simulink model "BalekaTorqueRamp"  (R2025a)
settings: Solver=FixedStepAuto  StartTime=0.0  StopTime=StopTime  RelTol=1e-3
values from neighbouring files (symbols this model uses):
  StopTime = 15    [StepParams.m]
undefined symbols (not defined in the file or in its folder): HS, IO291
libraries: aru_toolbox x7, simulink x4, speedgoatlib_IO691 x3, speedgoatlib_IO291 x1
settings Model: SimulationMode=external  Creator=Blue Fifth  LastModifiedBy=user
settings SolverCC: ConcurrentTasks=on  PositivePriorityOrder=on
settings OptimizationCC: BlockReduction=off  OptimizeBlockIOStorage=off
settings DebuggingCC: TasksWithSamePriorityMsg=none
settings HardwareCC: ProdBitPerLong=64.0  ProdLongLongMode=on  ProdHWDeviceType=Intel->x86-64 (Linux 64)
settings RTWCC: SystemTargetFile=speedgoat.tlc  TemplateMakefile=slrealtime_default_tmf  Toolchain=Simulink Real-Time Toolchain  BuildConfiguration=Faster Runs  CodeExecutionProfiling=on  TargetLang=C++  GPUComputeCapability=3.5  Description=Speedgoat Real-Time Target Machine
settings SimulinkRealTimeTargetCC: SLRTFileLogMaxRuns=1.0  ExtModeMaxTrigDuration=10.0  ExtModeStaticAllocSize=1000000.0  ExtModeTransport=0.0  MultiwordLength=2048.0  DynamicStringBufferSize=256.0  PreserveMATLABNamespacesInGeneratedCode=on  SubcomponentCodeInterfacePackaging=Reusable function  InstructionSetFMA=off  LogToMDFFile=off

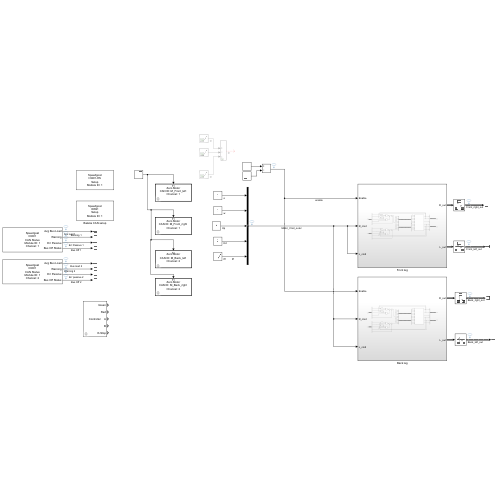
[thumbnail: Simulink's stored preview of the top-level diagram]
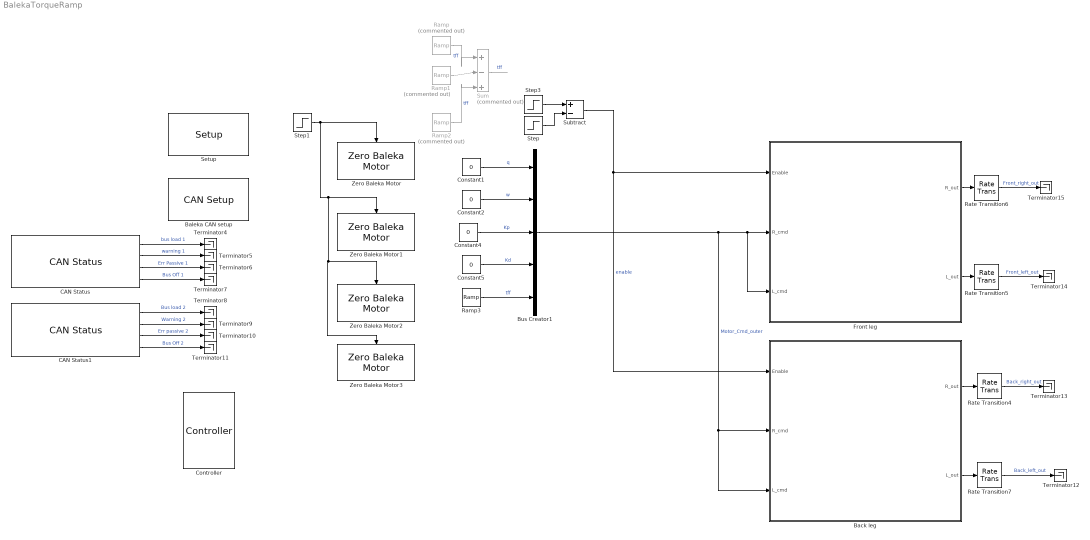
== system BalekaTorqueRamp ==
  Back leg : Subsystem
  Baleka CAN setup : speedgoatlib_IO691/Legacy/CAN Setup   moduletype=IO691  id=1  pciSlot=-1  chn1=CAN (HS)  chn2=CAN (HS)  chn3=Disabled  chn4=Disabled  initStruct=[]  termStruct=[struct('Channel',1,'Protocol','CAN','BRS',0,'Type','Extended','Identifier',1,'Data',[255, 255, 255, 255, 255, 255, 255, 253],'Pause',0.001), struct('Channel',2,'Protocol','CAN','BRS',0,'Type','Extended','Identifier',2,'Data',[255, 255, 255, 255, 255, 255, 255, 253],'Pause',0.001)]  ArbitrationbdrChn1=1.0 MBaud  ArbitrationManbdrChn1=[2,8,31,8]  FdbdrChn1=1.0 MBaud  FdManbdrChn1=[2,8,31,8]  ArbitrationbdrChn2=1.0 MBaud  ArbitrationManbdrChn2=[2,8,31,8]  FdbdrChn2=1.0 MBaud  FdManbdrChn2=[2,8,31,8]  ArbitrationbdrChn3=1.0 MBaud  ArbitrationManbdrChn3=[2,8,31,8]  FdbdrChn3=5.0 MBaud  FdManbdrChn3=[2,2,5,2]  ArbitrationbdrChn4=1.0 MBaud  ArbitrationManbdrChn4=[2,8,31,8]  FdbdrChn4=5.0 MBaud  FdManbdrChn4=[2,2,5,2]  moduleInitValues=[691 1 -1 -1]
      settings: SourceProductName=IO691
  Bus Creator1 : BusCreator  Inputs=5  OutDataTypeStr=Bus: MotorCmd  NonVirtualBus=on
      settings: InheritFromInputs=off
  CAN Status : speedgoatlib_IO691/Legacy/CAN Status  moduleId=1  sampleTime=0.001  channel=1  busRecovery=Auto  arrayOutput=off  controllerCpuLoad=off  controllerLiveCount=off  initModeAct=off  avgBusLoad=on  receiving=off  RxQueueEmpty=off  dataOverrunRcv=off  rxBufferLevel=off  txPending=off  dataOverrunTx=off  txBufferLevel=off  errWarnLimit=on  errPassLimit=on  errBusOff=on  busRecoveryCounter=off  busCouplingErr=off  transceiverErr=off  opMode=off  brp=off  timeSegment1=off  timeSegment2=off  synchronisationJumpWidth=off  dataTSEG1=off  dataTSEG2=off  dataSJW=off  moduleType=691  qtyStatBlk=1  ptIdx=0  isFDMod=0
      settings: SourceProductName=IO691
  CAN Status1 : speedgoatlib_IO691/Legacy/CAN Status  moduleId=1  sampleTime=0.001  channel=2  busRecovery=Auto  arrayOutput=off  controllerCpuLoad=off  controllerLiveCount=off  initModeAct=off  avgBusLoad=on  receiving=off  RxQueueEmpty=off  dataOverrunRcv=off  rxBufferLevel=off  txPending=off  dataOverrunTx=off  txBufferLevel=off  errWarnLimit=on  errPassLimit=on  errBusOff=on  busRecoveryCounter=off  busCouplingErr=off  transceiverErr=off  opMode=off  brp=off  timeSegment1=off  timeSegment2=off  synchronisationJumpWidth=off  dataTSEG1=off  dataTSEG2=off  dataSJW=off  moduleType=691  qtyStatBlk=1  ptIdx=0  isFDMod=0
      settings: SourceProductName=IO691
  Constant{1..2,4..5} (4 alike) : Constant  Value=0
  Controller : aru_toolbox/Controller
      settings: SourceProductName=ARU Toolbox
  Front leg : Subsystem
  Ramp : simulink/Sources/Ramp  Commented=on  slope=0.05  start=10  InitialOutput=0
  Ramp1 : simulink/Sources/Ramp  Commented=on  slope=0.1  start=40  InitialOutput=0
  Ramp2 : simulink/Sources/Ramp  Commented=on  slope=0.1  start=100  InitialOutput=0
  Ramp3 : simulink/Sources/Ramp  slope=0.05  start=5  InitialOutput=0
  Rate Transition{4..7} (4 alike) : RateTransition  OutPortSampleTime=1/1000
  "Setup " : speedgoatlib_IO291/Setup   parInternalModuleId=1  parPciSlot=-1  parModuleId=1  parModuleType=IO291-HS  parTtlDoChannels=[]  parTtlDoInitValues=1  parTtlDoReset=1  parTtlDiChannels=[1 2 3 4 5]  parIsolDiChannels=[]  parFetDoChannels=[1 2 3 4]  parFetDoInitValues=0  parFetDoReset=1
      settings: SourceProductName=IO291
  Step : Step  Time=StopTime-4  SampleTime=0
  Step1 : Step  Time=2  SampleTime=0
  Step3 : Step  SampleTime=0
  Subtract : Sum  Inputs=+-
  Sum : Sum  Commented=on  Inputs=|+-+
  Terminator{4..15} (12 alike) : Terminator
  Zero Baleka Motor : aru_toolbox/Baleka 2.5/Zero Baleka Motor  CAN_ID=M_Front_left  channel=1
      settings: SourceProductName=ARU Toolbox
  Zero Baleka Motor1 : aru_toolbox/Baleka 2.5/Zero Baleka Motor  CAN_ID=M_Front_right  channel=1
      settings: SourceProductName=ARU Toolbox
  Zero Baleka Motor2 : aru_toolbox/Baleka 2.5/Zero Baleka Motor  CAN_ID=M_Back_left  channel=2
      settings: SourceProductName=ARU Toolbox
  Zero Baleka Motor3 : aru_toolbox/Baleka 2.5/Zero Baleka Motor  CAN_ID=M_Back_right  channel=2
      settings: SourceProductName=ARU Toolbox
  wires:
  Step/1 -> Subtract/2
  Step3/1 -> Subtract/1
  Subtract/1 -> Back leg/1(Enable), Front leg/1(Enable)  "enable"
  Step1/1 -> Zero Baleka Motor3/Trigger, Zero Baleka Motor2/Trigger, Zero Baleka Motor1/Trigger, Zero Baleka Motor/Trigger
  CAN Status/1 -> Terminator4/1  "bus load 1"
  CAN Status/2 -> Terminator5/1  "warning 1"
  CAN Status/3 -> Terminator6/1  "Err Passive 1"
  CAN Status/4 -> Terminator7/1  "Bus Off 1"
  CAN Status1/1 -> Terminator8/1  "Bus load 2"
  CAN Status1/2 -> Terminator9/1  "Warning 2"
  CAN Status1/3 -> Terminator10/1  "Err passive 2"
  CAN Status1/4 -> Terminator11/1  "Bus Off 2"
  Constant1/1 -> Bus Creator1/1  "q"
  Constant2/1 -> Bus Creator1/2  "w"
  Constant4/1 -> Bus Creator1/3  "Kp"
  Constant5/1 -> Bus Creator1/4  "Kd"
  Bus Creator1/1 -> Back leg/3(L_cmd), Back leg/2(R_cmd), Front leg/3(L_cmd), Front leg/2(R_cmd)  "Motor_Cmd_outer"
  Ramp1/1 -> Sum/2
  Ramp2/1 -> Sum/3  "tff"
  Sum/1 -> ?  "tff"
  Ramp/1 -> Sum/1  "tff"
  Ramp3/1 -> Bus Creator1/5  "tff"
  Front leg/2(L_out) -> Rate Transition5/1
  Rate Transition7/1 -> Terminator12/1  "Back_left_out"
  Rate Transition4/1 -> Terminator13/1  "Back_right_out"
  Rate Transition6/1 -> Terminator15/1  "Front_right_out"
  Back leg/1(R_out) -> Rate Transition4/1
  Rate Transition5/1 -> Terminator14/1  "Front_left_out"
  Front leg/1(R_out) -> Rate Transition6/1
  Back leg/2(L_out) -> Rate Transition7/1

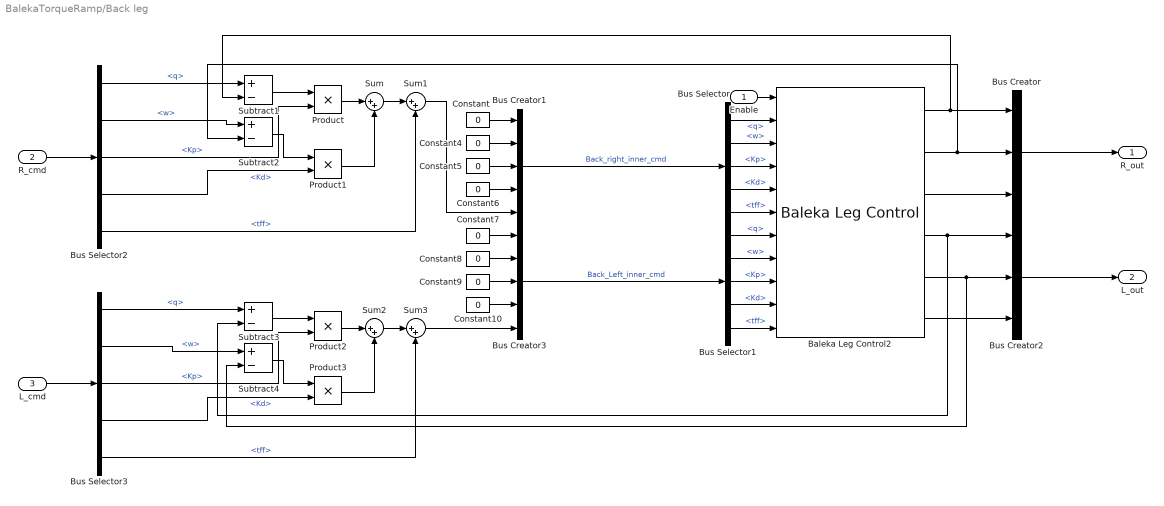
== system BalekaTorqueRamp/Back leg ==
  Enable : Inport
  R_cmd : Inport  Port=2
  L_cmd : Inport  Port=3
  Baleka Leg Control2 : aru_toolbox/Baleka 2.5/Baleka Leg Control  CAN_ID_L=M_Back_left  CAN_ID_R=M_Back_right  channel=2  Comm_freq=1000  enableOffsets=off  KtuneL=M_BL_torque  KtuneR=M_BR_torque
      settings: SourceProductName=ARU Toolbox
  Bus Creator : BusCreator  Inputs=3  OutDataTypeStr=Bus: MotorState  NonVirtualBus=on
      settings: InheritFromInputs=off
  Bus Creator1 : BusCreator  Inputs=5  OutDataTypeStr=Bus: MotorCmd  NonVirtualBus=on
      settings: InheritFromInputs=off
  Bus Creator2 : BusCreator  Inputs=3  OutDataTypeStr=Bus: MotorState  NonVirtualBus=on
      settings: InheritFromInputs=off
  Bus Creator3 : BusCreator  Inputs=5  OutDataTypeStr=Bus: MotorCmd  NonVirtualBus=on
      settings: InheritFromInputs=off
  Bus Selector{,1..3} (4 alike) : BusSelector  OutputSignals=q,w,Kp,Kd,tff
  Constant{,4..10} (8 alike) : Constant  Value=0
  Product{,1..3} (4 alike) : Product
  Subtract{1..4} (4 alike) : Sum  Inputs=+-
  Sum{,1..3} (4 alike) : Sum  Inputs=|++
  R_out : Outport
  L_out : Outport  Port=2
  wires:
  L_cmd/1 -> Bus Selector3/1
  R_cmd/1 -> Bus Selector2/1
  Product2/1 -> Sum2/1
  Product3/1 -> Sum2/2
  Subtract3/1 -> Product2/1
  Bus Selector3/2 -> Subtract4/1  "<w>"
  Subtract4/1 -> Product3/1
  Bus Selector3/3 -> Product2/2  "<Kp>"
  Bus Selector3/1 -> Subtract3/1  "<q>"
  Bus Selector3/4 -> Product3/2  "<Kd>"
  Bus Selector3/5 -> Sum3/2  "<tff>"
  Sum2/1 -> Sum3/1
  Bus Selector2/5 -> Sum1/2  "<tff>"
  Bus Selector2/4 -> Product1/2  "<Kd>"
  Subtract2/1 -> Product1/1
  Bus Selector2/2 -> Subtract2/1  "<w>"
  Product/1 -> Sum/1
  Bus Selector2/3 -> Product/2  "<Kp>"
  Bus Creator2/1 -> L_out/1
  Sum1/1 -> Bus Creator1/5
  Sum3/1 -> Bus Creator3/5
  Bus Creator/1 -> R_out/1
  Constant8/1 -> Bus Creator3/2
  Baleka Leg Control2/1 -> Bus Creator/1, Subtract1/2
  Constant7/1 -> Bus Creator3/1
  Bus Selector/3 -> Baleka Leg Control2/4  "<Kp>"
  Bus Selector1/5 -> Baleka Leg Control2/11  "<tff>"
  Subtract1/1 -> Product/1
  Constant6/1 -> Bus Creator1/4
  Baleka Leg Control2/6 -> Bus Creator2/3
  Bus Selector2/1 -> Subtract1/1  "<q>"
  Bus Selector/1 -> Baleka Leg Control2/2  "<q>"
  Sum/1 -> Sum1/1
  Baleka Leg Control2/5 -> Subtract4/2, Bus Creator2/2
  Bus Creator1/1 -> Bus Selector/1  "Back_right_inner_cmd"
  Bus Creator3/1 -> Bus Selector1/1  "Back_Left_inner_cmd"
  Baleka Leg Control2/2 -> Bus Creator/2, Subtract2/2
  Constant4/1 -> Bus Creator1/2
  Constant10/1 -> Bus Creator3/4
  Bus Selector1/3 -> Baleka Leg Control2/9  "<Kp>"
  Bus Selector1/1 -> Baleka Leg Control2/7  "<q>"
  Bus Selector/5 -> Baleka Leg Control2/6  "<tff>"
  Bus Selector/2 -> Baleka Leg Control2/3  "<w>"
  Bus Selector1/4 -> Baleka Leg Control2/10  "<Kd>"
  Product1/1 -> Sum/2
  Constant9/1 -> Bus Creator3/3
  Constant/1 -> Bus Creator1/1
  Baleka Leg Control2/4 -> Subtract3/2, Bus Creator2/1
  Bus Selector1/2 -> Baleka Leg Control2/8  "<w>"
  Baleka Leg Control2/3 -> Bus Creator/3
  Enable/1 -> Baleka Leg Control2/1
  Constant5/1 -> Bus Creator1/3
  Bus Selector/4 -> Baleka Leg Control2/5  "<Kd>"

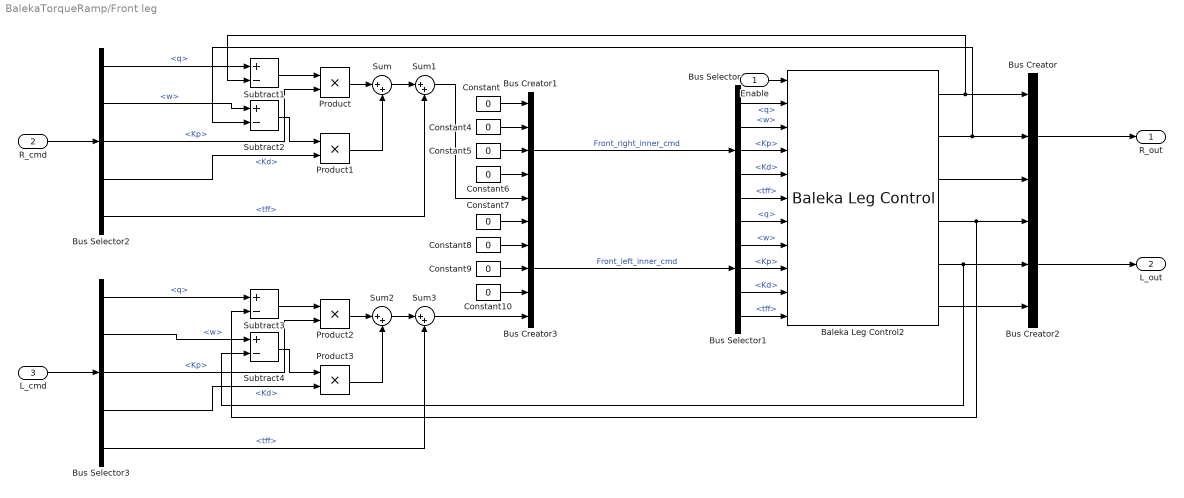
== system BalekaTorqueRamp/Front leg ==
  Enable : Inport
  R_cmd : Inport  Port=2
  L_cmd : Inport  Port=3
  Baleka Leg Control2 : aru_toolbox/Baleka 2.5/Baleka Leg Control  CAN_ID_L=M_Front_left  CAN_ID_R=M_Front_right  channel=1  Comm_freq=1000  enableOffsets=off  KtuneL=M_FL_torque  KtuneR=M_FR_torque
      settings: SourceProductName=ARU Toolbox
  Bus Creator : BusCreator  Inputs=3  OutDataTypeStr=Bus: MotorState  NonVirtualBus=on
      settings: InheritFromInputs=off
  Bus Creator1 : BusCreator  Inputs=5  OutDataTypeStr=Bus: MotorCmd  NonVirtualBus=on
      settings: InheritFromInputs=off
  Bus Creator2 : BusCreator  Inputs=3  OutDataTypeStr=Bus: MotorState  NonVirtualBus=on
      settings: InheritFromInputs=off
  Bus Creator3 : BusCreator  Inputs=5  OutDataTypeStr=Bus: MotorCmd  NonVirtualBus=on
      settings: InheritFromInputs=off
  Bus Selector{,1..3} (4 alike) : BusSelector  OutputSignals=q,w,Kp,Kd,tff
  Constant{,4..10} (8 alike) : Constant  Value=0
  Product{,1..3} (4 alike) : Product
  Subtract{1..4} (4 alike) : Sum  Inputs=+-
  Sum{,1..3} (4 alike) : Sum  Inputs=|++
  R_out : Outport
  L_out : Outport  Port=2
  wires:
  Bus Selector/4 -> Baleka Leg Control2/5  "<Kd>"
  Constant5/1 -> Bus Creator1/3
  Enable/1 -> Baleka Leg Control2/1
  Baleka Leg Control2/3 -> Bus Creator/3
  Bus Selector1/2 -> Baleka Leg Control2/8  "<w>"
  Baleka Leg Control2/4 -> Subtract3/2, Bus Creator2/1
  Constant/1 -> Bus Creator1/1
  Constant9/1 -> Bus Creator3/3
  Product1/1 -> Sum/2
  Bus Selector1/4 -> Baleka Leg Control2/10  "<Kd>"
  Bus Selector/2 -> Baleka Leg Control2/3  "<w>"
  Bus Selector/5 -> Baleka Leg Control2/6  "<tff>"
  Bus Selector1/1 -> Baleka Leg Control2/7  "<q>"
  Bus Selector1/3 -> Baleka Leg Control2/9  "<Kp>"
  Constant10/1 -> Bus Creator3/4
  Constant4/1 -> Bus Creator1/2
  Baleka Leg Control2/2 -> Subtract2/2, Bus Creator/2
  Bus Creator3/1 -> Bus Selector1/1  "Front_left_inner_cmd"
  Bus Creator1/1 -> Bus Selector/1  "Front_right_inner_cmd"
  Baleka Leg Control2/5 -> Subtract4/2, Bus Creator2/2
  Sum/1 -> Sum1/1
  Bus Selector/1 -> Baleka Leg Control2/2  "<q>"
  Bus Selector2/1 -> Subtract1/1  "<q>"
  Baleka Leg Control2/6 -> Bus Creator2/3
  Constant6/1 -> Bus Creator1/4
  Subtract1/1 -> Product/1
  Bus Selector1/5 -> Baleka Leg Control2/11  "<tff>"
  Bus Selector/3 -> Baleka Leg Control2/4  "<Kp>"
  Constant7/1 -> Bus Creator3/1
  Baleka Leg Control2/1 -> Subtract1/2, Bus Creator/1
  Constant8/1 -> Bus Creator3/2
  Bus Creator/1 -> R_out/1
  Sum3/1 -> Bus Creator3/5
  Sum1/1 -> Bus Creator1/5
  Bus Creator2/1 -> L_out/1
  Bus Selector2/3 -> Product/2  "<Kp>"
  Product/1 -> Sum/1
  Bus Selector2/2 -> Subtract2/1  "<w>"
  Subtract2/1 -> Product1/1
  Bus Selector2/4 -> Product1/2  "<Kd>"
  Bus Selector2/5 -> Sum1/2  "<tff>"
  Sum2/1 -> Sum3/1
  Bus Selector3/5 -> Sum3/2  "<tff>"
  Bus Selector3/4 -> Product3/2  "<Kd>"
  Bus Selector3/1 -> Subtract3/1  "<q>"
  Bus Selector3/3 -> Product2/2  "<Kp>"
  Subtract4/1 -> Product3/1
  Bus Selector3/2 -> Subtract4/1  "<w>"
  Subtract3/1 -> Product2/1
  Product3/1 -> Sum2/2
  Product2/1 -> Sum2/1
  R_cmd/1 -> Bus Selector2/1
  L_cmd/1 -> Bus Selector3/1
